simulink model "Ex10_4_2_RelayControlledMotor"  (R2023a)
settings: Solver=VariableStepAuto  StartTime=0.0  StopTime=.1  RelTol=1e-3
settings Model: Creator=Norb  LastModifiedBy=Norb

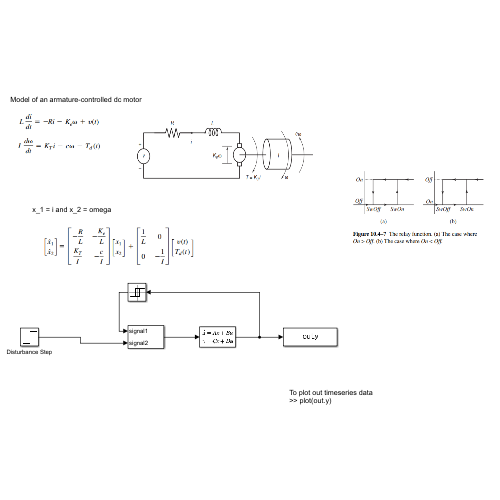
[thumbnail: Simulink's stored preview of the top-level diagram]
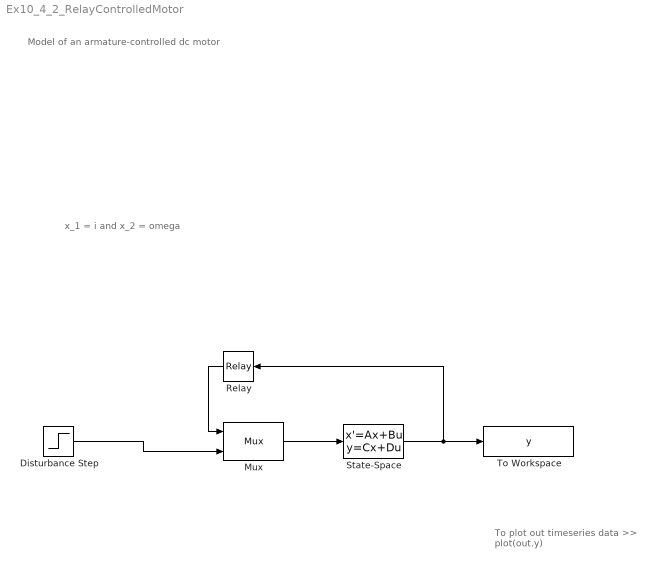
== system Ex10_4_2_RelayControlledMotor ==
  note: To plot out timeseries data
      | >> plot(out.y)
  note: x_1 = i and x_2 = omega
  note: Model of an armature-controlled dc motor
  Disturbance Step : Step  Time=.05  After=3  SampleTime=0
  Mux : Mux  Inputs=2
      settings: DisplayOption=signals
  Relay : Relay  OnSwitchValue=350  OffSwitchValue=250  OnOutputValue=0  OffOutputValue=100
  State-Space : StateSpace  A=[-300,-20;666.7,-166.7]  B=[500,0; 0,-16667]  C=[0,1]  D=[0,0]  InitialCondition=0
  To Workspace : ToWorkspace  VariableName=y  SaveFormat=Timeseries  SampleTime=-1
  wires:
  Disturbance Step/1 -> Mux/2
  Relay/1 -> Mux/1
  Mux/1 -> State-Space/1
  State-Space/1 -> To Workspace/1, Relay/1
